simulink model "Energiebedarf_Mod_WLTC"  (R2018a)
settings: Solver=ode4  StartTime=0.0  StopTime=t_WLTC_s(end)  FixedStep=1  RelTol=1e-3  EnableMultiTasking=on
values from neighbouring files (symbols this model uses):
  cwA = 0.7    [Energiebedarf_single.m]
  etaRec = 0.5    [Energiebedarf_single.m]
  fR = 0.012    [Energiebedarf_single.m]
  g = 9.81    [Energiebedarf_single.m]
  m = 1500    [Energiebedarf_single.m]
  rho = 1.2    [Energiebedarf_single.m]
  t_WLTC_s = [0 1 2 3 4 5 6 7 8 9 10 11 ... (1801 elements, 1801x1)]    [WLTC.mat]
  v_WLTC_kph = [0 0 0 0 0 0 0 0 0 0 0 0 ... (1801 elements, 1801x1)]    [WLTC.mat]
libraries: simulink x2
settings Model: Creator=raschul  LastModifiedBy=raschul
settings DataIOCC: LimitDataPoints=on  SaveFormat=Array  SignalLoggingSaveFormat=ModelDataLogs
settings OptimizationCC: ExpressionDepthLimit=2147483647  LifeSpan=inf
settings DebuggingCC: UnderspecifiedInitializationDetection=Classic  MergeDetectMultiDrivingBlocksExec=none  SolverPrmCheckMsg=warning  FcnCallInpInsideContextMsg=warning  AllowSymbolicDim=off  StateNameClashWarn=warning  SFUnexpectedBacktrackingDiag=warning  SFNoUnconditionalDefaultTransitionDiag=warning  SFExecutionAtInitializationDiag=none
settings HardwareCC: ProdBitPerPointer=32  ProdBitPerSizeT=32  ProdBitPerPtrDiffT=32  ProdLargestAtomicFloat=None  ProdIntDivRoundTo=Undefined  ProdEndianess=Unspecified  ProdWordSize=32  ProdHWDeviceType=32-bit Generic
settings ModelReferenceCC: PropagateSignalLabelsOutOfModel=off
settings CodeAppCC: StateflowObjectComments=on
settings GRTTargetCC: TargetLangStandard=C89/C90 (ANSI)  GeneratePreprocessorConditionals=Disable all  CombineOutputUpdateFcns=off  GRTInterface=on
settings ConfigComp: CovMetricSettings=dw  CovHtmlReporting=on  CovSaveCumulativeToWorkspaceVar=on  CovSaveSingleToWorkspaceVar=on  CovExternalEMLEnable=off

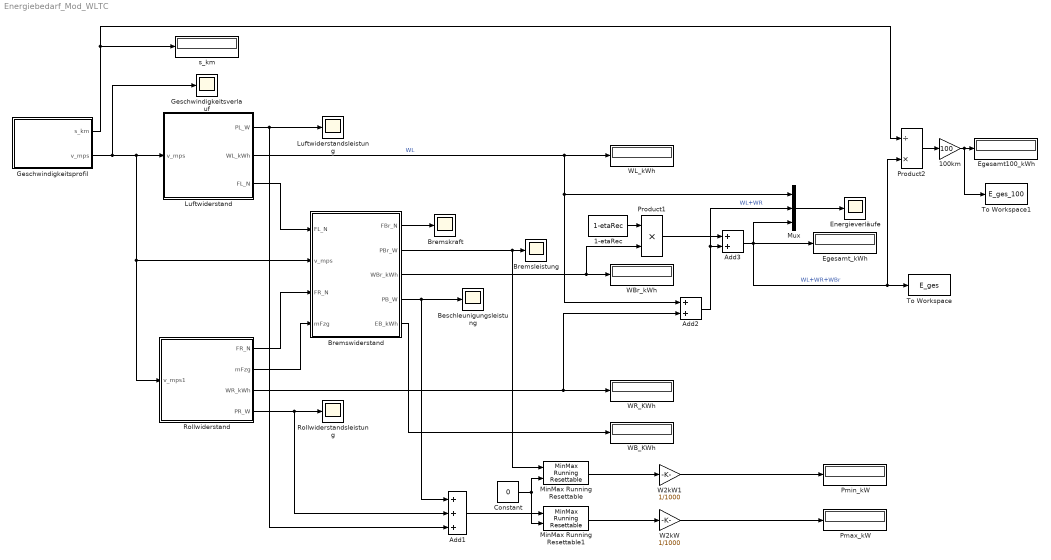
== system Energiebedarf_Mod_WLTC ==
  1-etaRec : Constant  Value=1-etaRec
  100km : Gain  Gain=100
  Add1 : Sum  Inputs=+++
  Add2 : Sum
  Add3 : Sum
  Beschleunigungsleistung : Scope
  Bremskraft : Scope
  Bremsleistung : Scope
  Bremswiderstand : Subsystem
  Constant : Constant  Value=0
  Egesamt100_kWh : Display
  Egesamt_kWh : Display
  Energieverläufe : Scope
  Geschwindigkeitsprofil : Subsystem
  Geschwindigkeitsverlauf : Scope
  Luftwiderstand : Subsystem
  Luftwiderstandsleistung : Scope
  MinMax Running Resettable : simulink/Math Operations/MinMax Running Resettable  Function=max  vinit=0.0
  MinMax Running Resettable1 : simulink/Math Operations/MinMax Running Resettable  Function=max  vinit=0.0
  Mux : Mux  Inputs=3
  Pmax_kW : Display
  Pmin_kW : Display
  Product1 : Product  RndMeth=Zero
  Product2 : Product  Inputs=/*  RndMeth=Zero
  Rollwiderstand : Subsystem
  Rollwiderstandsleistung : Scope
  To Workspace : ToWorkspace  VariableName=E_ges  SaveFormat=Timeseries  SampleTime=-1
  To Workspace1 : ToWorkspace  VariableName=E_ges_100  SaveFormat=Timeseries  SampleTime=-1
  W2kW : Gain  Gain=1/1000
  W2kW1 : Gain  Gain=1/1000
  WB_KWh : Display
  WBr_kWh : Display
  WL_kWh : Display
  WR_KWh : Display
  s_km : Display
  wires:
  Geschwindigkeitsprofil/2(v_mps) -> Geschwindigkeitsverlauf/1, Rollwiderstand/1(v_mps1), Bremswiderstand/2(v_mps), Luftwiderstand/1(v_mps)
  Luftwiderstand/2(WL_kWh) -> Mux/1, Add2/1, WL_kWh/1  "WL"
  Rollwiderstand/3(WR_kWh) -> Add2/2, WR_KWh/1
  Add2/1 -> Mux/2, Add3/2  "WL+WR"
  Add3/1 -> Product2/2, To Workspace/1, Mux/3, Egesamt_kWh/1  "WL+WR+WBr"
  Mux/1 -> Energieverläufe/1
  Luftwiderstand/1(PL_W) -> Add1/3, Luftwiderstandsleistung/1
  Luftwiderstand/3(FL_N) -> Bremswiderstand/1(FL_N)
  Rollwiderstand/4(PR_W) -> Add1/2, Rollwiderstandsleistung/1
  Rollwiderstand/1(FR_N) -> Bremswiderstand/3(FR_N)
  Rollwiderstand/2(mFzg) -> Bremswiderstand/4(mFzg)
  Bremswiderstand/1(FBr_N) -> Bremskraft/1
  Bremswiderstand/2(PBr_W) -> MinMax Running Resettable/1, Bremsleistung/1
  Geschwindigkeitsprofil/1(s_km) -> Product2/1, s_km/1
  Bremswiderstand/4(PB_W) -> Beschleunigungsleistung/1, Add1/1
  Add1/1 -> MinMax Running Resettable1/1
  MinMax Running Resettable1/1 -> W2kW/1
  W2kW/1 -> Pmax_kW/1
  MinMax Running Resettable/1 -> W2kW1/1
  W2kW1/1 -> Pmin_kW/1
  Constant/1 -> MinMax Running Resettable1/2, MinMax Running Resettable/2
  Product1/1 -> Add3/1
  Bremswiderstand/5(EB_kWh) -> WB_KWh/1
  1-etaRec/1 -> Product1/1
  Bremswiderstand/3(WBr_kWh) -> Product1/2, WBr_kWh/1
  Product2/1 -> 100km/1
  100km/1 -> To Workspace1/1, Egesamt100_kWh/1

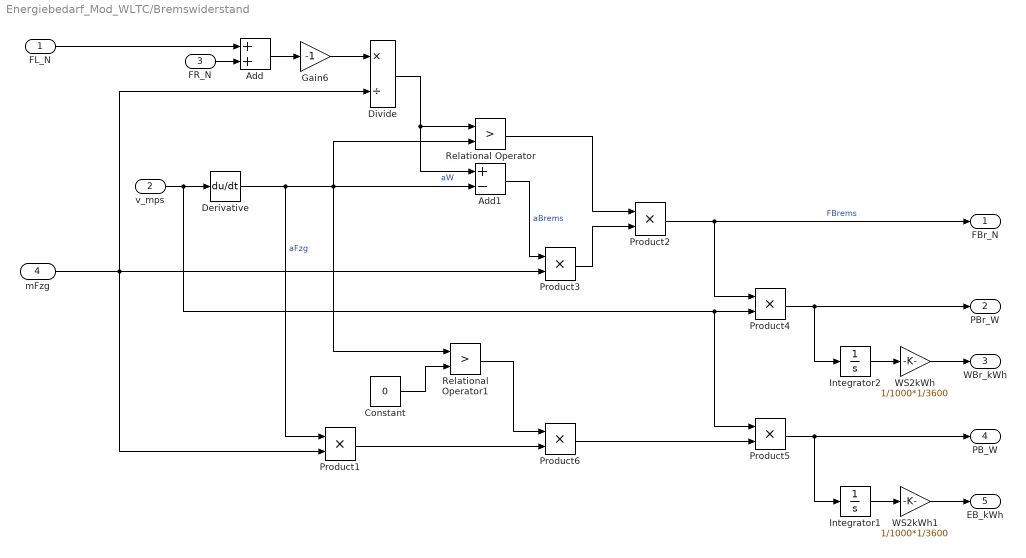
== system Energiebedarf_Mod_WLTC/Bremswiderstand ==
  FL_N : Inport
  v_mps : Inport  Port=2
  FR_N : Inport  Port=3
  mFzg : Inport  Port=4
  Add : Sum
  Add1 : Sum  Inputs=+-
  Constant : Constant  Value=0
  Derivative : Derivative
  Divide : Product  Inputs=*/
  Gain6 : Gain  Gain=-1
  Integrator1 : Integrator
  Integrator2 : Integrator
  Product{1..6} (6 alike) : Product  RndMeth=Zero
  Relational Operator : RelationalOperator  Operator=>  OutDataTypeStr=boolean  RndMeth=Nearest
  Relational Operator1 : RelationalOperator  Operator=>  OutDataTypeStr=boolean  RndMeth=Nearest
  WS2kWh : Gain  Gain=1/1000*1/3600
  WS2kWh1 : Gain  Gain=1/1000*1/3600
  FBr_N : Outport
  PBr_W : Outport  Port=2
  WBr_kWh : Outport  Port=3
  PB_W : Outport  Port=4
  EB_kWh : Outport  Port=5
  wires:
  Derivative/1 -> Product1/1, Relational Operator1/1, Relational Operator/2, Add1/2  "aFzg"
  Add/1 -> Gain6/1
  Gain6/1 -> Divide/1
  Divide/1 -> Add1/1, Relational Operator/1  "aW"
  Relational Operator/1 -> Product2/1
  Add1/1 -> Product3/1  "aBrems"
  Product3/1 -> Product2/2
  mFzg/1 -> Product1/2, Product3/2, Divide/2
  v_mps/1 -> Product5/1, Product4/2, Derivative/1
  FL_N/1 -> Add/1
  FR_N/1 -> Add/2
  Product2/1 -> Product4/1, FBr_N/1  "FBrems"
  Integrator2/1 -> WS2kWh/1
  Product4/1 -> PBr_W/1, Integrator2/1
  WS2kWh/1 -> WBr_kWh/1
  Constant/1 -> Relational Operator1/2
  Relational Operator1/1 -> Product6/1
  Product1/1 -> Product6/2
  Product6/1 -> Product5/2
  Integrator1/1 -> WS2kWh1/1
  Product5/1 -> Integrator1/1, PB_W/1
  WS2kWh1/1 -> EB_kWh/1

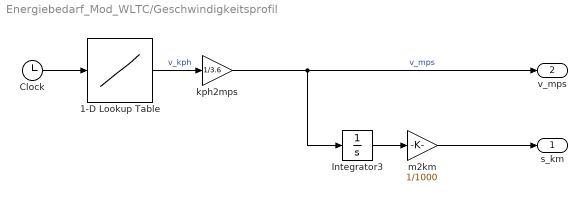
== system Energiebedarf_Mod_WLTC/Geschwindigkeitsprofil ==
  1-D Lookup Table : Lookup_n-D  NumberOfTableDimensions=1  BreakpointsForDimension1=t_WLTC_s  Table=v_WLTC_kph  RndMeth=Simplest  InputSameDT=on
  Clock : Clock
  Integrator3 : Integrator
  kph2mps : Gain  Gain=1/3.6
  m2km : Gain  Gain=1/1000
  s_km : Outport
  v_mps : Outport  Port=2
  wires:
  1-D Lookup Table/1 -> kph2mps/1  "v_kph"
  Clock/1 -> 1-D Lookup Table/1
  kph2mps/1 -> Integrator3/1, v_mps/1  "v_mps"
  Integrator3/1 -> m2km/1
  m2km/1 -> s_km/1

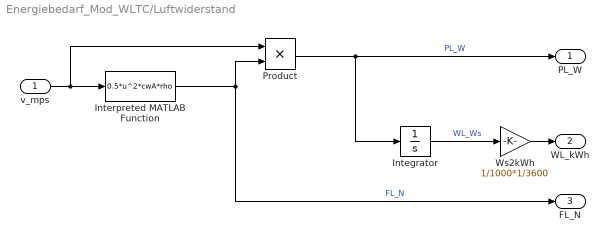
== system Energiebedarf_Mod_WLTC/Luftwiderstand ==
  v_mps : Inport
  Integrator : Integrator
  Interpreted MATLAB Function : MATLABFcn  MATLABFcn=0.5*u^2*cwA*rho
  Product : Product  RndMeth=Zero
  Ws2kWh : Gain  Gain=1/1000*1/3600
  PL_W : Outport
  WL_kWh : Outport  Port=2
  FL_N : Outport  Port=3
  wires:
  Interpreted MATLAB Function/1 -> Product/2, FL_N/1  "FL_N"
  Product/1 -> Integrator/1, PL_W/1  "PL_W"
  Integrator/1 -> Ws2kWh/1  "WL_Ws"
  v_mps/1 -> Product/1, Interpreted MATLAB Function/1
  Ws2kWh/1 -> WL_kWh/1

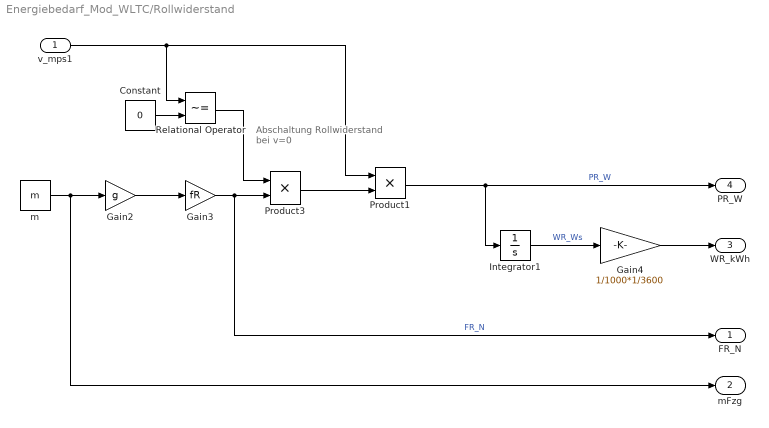
== system Energiebedarf_Mod_WLTC/Rollwiderstand ==
  note: Abschaltung
      | Rollwiderstand
      | bei v=0
  v_mps1 : Inport
  Constant : Constant  Value=0
  Gain2 : Gain  Gain=g
  Gain3 : Gain  Gain=fR
  Gain4 : Gain  Gain=1/1000*1/3600
  Integrator1 : Integrator
  Product1 : Product  RndMeth=Zero
  Product3 : Product  RndMeth=Zero
  Relational Operator : RelationalOperator  Operator=~=  OutDataTypeStr=boolean  RndMeth=Nearest
  m : Constant  Value=m
  FR_N : Outport
  mFzg : Outport  Port=2
  WR_kWh : Outport  Port=3
  PR_W : Outport  Port=4
  wires:
  m/1 -> Gain2/1, mFzg/1
  Gain2/1 -> Gain3/1
  Product1/1 -> Integrator1/1, PR_W/1  "PR_W"
  Integrator1/1 -> Gain4/1  "WR_Ws"
  Gain4/1 -> WR_kWh/1
  Relational Operator/1 -> Product3/1
  v_mps1/1 -> Product1/1, Relational Operator/1
  Constant/1 -> Relational Operator/2
  Gain3/1 -> Product3/2, FR_N/1  "FR_N"
  Product3/1 -> Product1/2
